simulink model "p1"  (R2020b)
settings: Solver=VariableStepAuto  StartTime=0.0  StopTime=10  RelTol=1e-3
undefined symbols (not defined in the file): A, A1, B, B1, C, C1, K, K1, KDelay, L
settings Model: Creator=Julian  LastModifiedBy=Julian

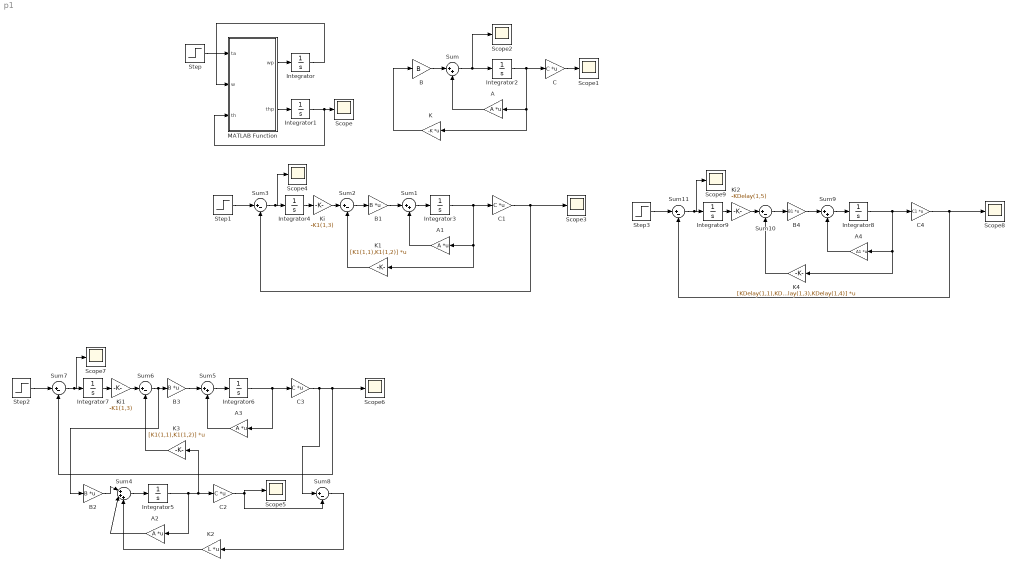
== system p1 ==
  A{,1..3} (4 alike) : Gain  Gain=A  Multiplication=Matrix(K*u)
  A4 : Gain  Gain=A1  Multiplication=Matrix(K*u)
  B : Gain  Gain=B
  B1 : Gain  Gain=B  Multiplication=Matrix(K*u)
  B2 : Gain  Gain=B  Multiplication=Matrix(K*u)
  B3 : Gain  Gain=B  Multiplication=Matrix(K*u)
  B4 : Gain  Gain=B1  Multiplication=Matrix(K*u)
  C{,1..3} (4 alike) : Gain  Gain=C  Multiplication=Matrix(K*u)
  C4 : Gain  Gain=C1  Multiplication=Matrix(K*u)
  Integrator{,1,3..9} (9 alike) : Integrator
  Integrator2 : Integrator  InitialCondition=1
  K : Gain  Gain=-K  Multiplication=Matrix(K*u)
  K1 : Gain  Gain=[K1(1,1),K1(1,2)]  Multiplication=Matrix(K*u)
  K2 : Gain  Gain=L  Multiplication=Matrix(K*u)
  K3 : Gain  Gain=[K1(1,1),K1(1,2)]  Multiplication=Matrix(K*u)
  K4 : Gain  Gain=[KDelay(1,1),KDelay(1,2),KDelay(1,3),KDelay(1,4)]  Multiplication=Matrix(K*u)
  Ki : Gain  Gain=-K1(1,3)
  Ki1 : Gain  Gain=-K1(1,3)
  Ki2 : Gain  Gain=-KDelay(1,5)
  MATLAB Function : MATLAB Function  TreatAsAtomicUnit=on
  Scope{,1..9} (10 alike) : Scope
  Step : Step  SampleTime=0
  Step1 : Step  SampleTime=0
  Step2 : Step  Time=0  SampleTime=0
  Step3 : Step  Time=0  SampleTime=0
  Sum{,1,5,9} (4 alike) : Sum  Inputs=|++
  Sum{2..3,6..8,10..11} (7 alike) : Sum  Inputs=|+-
  Sum4 : Sum  Inputs=|+++
  wires:
  Step/1 -> MATLAB Function/1(ta)
  MATLAB Function/2(thp) -> Integrator1/1
  MATLAB Function/1(wp) -> Integrator/1
  Integrator/1 -> MATLAB Function/2(w)
  Integrator1/1 -> Scope/1, MATLAB Function/3(th)
  B/1 -> Sum/1
  Sum/1 -> Scope2/1, Integrator2/1
  Integrator2/1 -> C/1, K/1, A/1
  A/1 -> Sum/2
  K/1 -> B/1
  C/1 -> Scope1/1
  A1/1 -> Sum1/2
  Sum1/1 -> Integrator3/1
  B1/1 -> Sum1/1
  Integrator3/1 -> C1/1, K1/1, A1/1
  Sum2/1 -> B1/1
  K1/1 -> Sum2/2
  Sum3/1 -> Scope4/1, Integrator4/1
  Step1/1 -> Sum3/1
  Ki/1 -> Sum2/1
  Integrator4/1 -> Ki/1
  Sum4/1 -> Integrator5/1
  B2/1 -> Sum4/1
  Integrator5/1 -> K3/1, C2/1, A2/1
  A2/1 -> Sum4/2
  K2/1 -> Sum4/3
  Integrator7/1 -> Ki1/1
  Sum5/1 -> Integrator6/1
  Ki1/1 -> Sum6/1
  K3/1 -> Sum6/2
  B3/1 -> Sum5/1
  Step2/1 -> Sum7/1
  Integrator6/1 -> C3/1, A3/1
  C3/1 -> Sum8/1, Scope6/1, Sum7/2
  A3/1 -> Sum5/2
  Sum7/1 -> Scope7/1, Integrator7/1
  Sum6/1 -> B2/1, B3/1
  C2/1 -> Sum8/2, Scope5/1
  Sum8/1 -> K2/1
  C1/1 -> Scope3/1, Sum3/2
  Sum11/1 -> Scope9/1, Integrator9/1
  Step3/1 -> Sum11/1
  Ki2/1 -> Sum10/1
  C4/1 -> Scope8/1, Sum11/2
  Sum9/1 -> Integrator8/1
  A4/1 -> Sum9/2
  K4/1 -> Sum10/2
  Integrator9/1 -> Ki2/1
  Integrator8/1 -> C4/1, K4/1, A4/1
  B4/1 -> Sum9/1
  Sum10/1 -> B4/1

== matlab function p1/MATLAB Function ==
  data: ta input; wp output; w input; th input; thp output
function [wp,thp] = fcn(ta,w,th)
m=1;
g=9.81;
l=0.1;
a=l/2;
k=0.1;

thp=w;
wp=(1/(m*l^2))*(ta-2*k*a*a*(-sin(th)*sin(th)+cos(th)*cos(th))-l*m*g*sin(th));
